simulink model "gm_sampleModel2052_3_sub"  (R2023a)
settings: Solver=VariableStepAuto  StartTime=0.0  StopTime=10.0  RelTol=1e-3
libraries: simulink x5, hdlsllib x1
settings Model: Creator=user1  LastModifiedBy=user1
settings OptimizationCC: BlockReduction=off  ConditionallyExecuteInputs=off
settings DebuggingCC: InheritedTsInSrcMsg=none

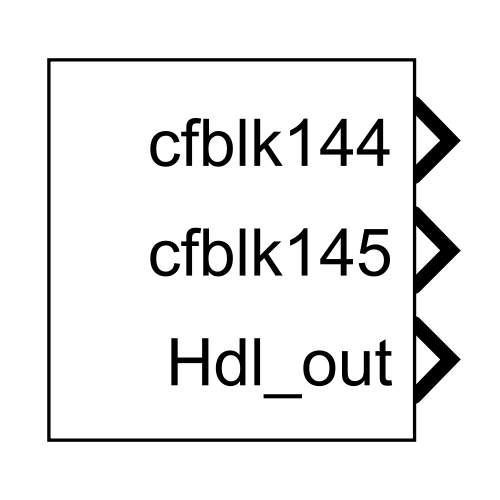
[thumbnail: Simulink's stored preview of the top-level diagram]
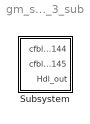
== system gm_sampleModel2052_3_sub ==
  Subsystem : Subsystem

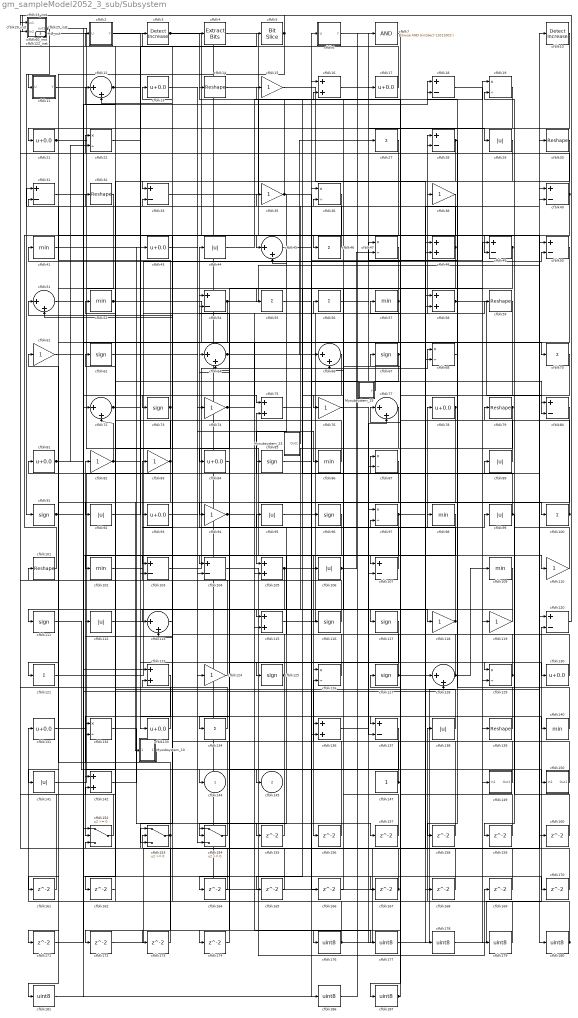
== system gm_sampleModel2052_3_sub/Subsystem ==
  Mysubsystem_10 : Subsystem
  Mysubsystem_15 : Subsystem
  Mysubsystem_23 : Subsystem
  cfblk10 : simulink/Logic and Bit Operations/Detect Increase  vinit=0.0  OutDataTypeStr=uint8
      settings: LibrarySourceBlock=|
      | hdlsllib/Logic and Bit
      | Operations/Detect
      | Increase
  cfblk{27,46,55..56,70,100,121,134} (8 alike) : Sum  Inputs=+  OutDataTypeStr=uint8
  cfblk{14,30,32,59,79,101,139} (7 alike) : Reshape
  cfblk{41,52,57,86,98,102,109,140} (8 alike) : MinMax  OutDataTypeStr=uint8
  cfblk{18,28,31,33,40,49..50,54,80,103..104,107,120,137} (14 alike) : Sum  Inputs=+-  OutDataTypeStr=uint8
  cfblk{16,48,58,75,105,115,123,136,142} (9 alike) : Sum  OutDataTypeStr=uint8
  cfblk{29,44,89,92,95,99,106,112,138,141} (10 alike) : Abs  OutDataTypeStr=uint8  SaturateOnIntegerOverflow=off
  cfblk108_inst : Subsystem
  cfblk11 : Subsystem  mask(Detect Fall Nonpositive){vinit=double(0), InputProcessing=Elements as channels (sample based), OutDataTypeStr=uint8}
      mask prompts: vinit "Simulink:masks:InitialCondition_MP"; InputProcessing "Simulink:masks:InputProcessing_MP"; OutDataTypeStr "Simulink:masks:OutputDataType_MP"
      mask help: Simulink:masks:DetectFallNonpositive_MD
      mask init:
      | InputProcessing = 'Elements as channels (sample based)';
      | OutDataTypeStr = 'uint8';
      | vinit = double(0);
      mask TypeOptions InputProcessing: Simulink:masks:ColumnsAsChannelsFrameBased | Simulink:masks:ElementsAsChannelsSampleBased
      mask TypeOptions OutDataTypeStr: Simulink:masks:uint8 | Simulink:masks:boolean
      mask Display: fprintf('U <= 0\n&  NOT\nU/z <= 0')
  cfblk{15,35,38,61,74,76,82..83,94,110,118..119,124} (13 alike) : Gain  OutDataTypeStr=uint8
  cfblk{62,67,73,85,91,96,111,116..117,125,127} (11 alike) : Signum
  cfblk{12,45,51,64,66,72,77,113,128} (9 alike) : Sum  Inputs=|++  OutDataTypeStr=uint8
  cfblk122_inst : Subsystem
  cfblk{19,22,36,47,68,87,97,126,129,132} (10 alike) : Product  Inputs=*/  OutDataTypeStr=uint8  RndMeth=Zero  SaturateOnIntegerOverflow=on
  cfblk{13,17,21,43,78,81,84,93,130..131,133} (11 alike) : Bias  Bias=0.0  SaturateOnIntegerOverflow=off
  cfblk147 : Constant  OutDataTypeStr=uint8  SampleTime=-1
  cfblk149 : Subsystem
  cfblk150 : Subsystem
  cfblk152 : Switch  OutDataTypeStr=uint8  SaturateOnIntegerOverflow=off  InputSameDT=off
  cfblk153 : Switch  OutDataTypeStr=uint8  SaturateOnIntegerOverflow=off  InputSameDT=off
  cfblk154 : Switch  OutDataTypeStr=uint8  SaturateOnIntegerOverflow=off  InputSameDT=off
  cfblk{155..162,164..174} (19 alike) : Delay  SampleTime=1
  cfblk{176..181,186..187} (8 alike) : DataTypeConversion  OutDataTypeStr=uint8  SaturateOnIntegerOverflow=off  RndMeth=Floor
  cfblk2 : Subsystem  mask(Detect Fall Nonpositive){vinit=double(0), InputProcessing=Elements as channels (sample based), OutDataTypeStr=uint8}
      mask prompts: vinit "Simulink:masks:InitialCondition_MP"; InputProcessing "Simulink:masks:InputProcessing_MP"; OutDataTypeStr "Simulink:masks:OutputDataType_MP"
      mask help: Simulink:masks:DetectFallNonpositive_MD
      mask init:
      | InputProcessing = 'Elements as channels (sample based)';
      | OutDataTypeStr = 'uint8';
      | vinit = double(0);
      mask TypeOptions InputProcessing: Simulink:masks:ColumnsAsChannelsFrameBased | Simulink:masks:ElementsAsChannelsSampleBased
      mask TypeOptions OutDataTypeStr: Simulink:masks:uint8 | Simulink:masks:boolean
      mask Display: fprintf('U <= 0\n&  NOT\nU/z <= 0')
  cfblk20_inst : Subsystem
  cfblk23_inst : Subsystem
  cfblk25_inst : Subsystem
  cfblk3 : simulink/Logic and Bit Operations/Detect Increase  vinit=0.0  OutDataTypeStr=uint8
      settings: LibrarySourceBlock=|
      | hdlsllib/Logic and Bit
      | Operations/Detect
      | Increase
  cfblk4 : simulink/Logic and Bit Operations/Extract Bits  bitsToExtract=Upper half  numBits=8  bitIdxRange=[0 7]  outScalingMode=Preserve fixed-point scaling
      settings: LibrarySourceBlock=|
      | hdlsllib/Logic and Bit
      | Operations/Extract Bits
  cfblk5 : hdlsllib/Logic and Bit Operations/Bit Slice  lidx=7  ridx=0
  cfblk6 : Subsystem  mask(Detect Rise Nonnegative){vinit=double(0), InputProcessing=Elements as channels (sample based), OutDataTypeStr=uint8}
      mask prompts: vinit "Simulink:masks:InitialCondition_MP"; InputProcessing "Simulink:masks:InputProcessing_MP"; OutDataTypeStr "Simulink:masks:OutputDataType_MP"
      mask help: Simulink:masks:DetectRiseNonnegative_MD
      mask init:
      | InputProcessing = 'Elements as channels (sample based)';
      | OutDataTypeStr = 'uint8';
      | vinit = double(0);
      mask TypeOptions InputProcessing: Simulink:masks:ColumnsAsChannelsFrameBased | Simulink:masks:ElementsAsChannelsSampleBased
      mask TypeOptions OutDataTypeStr: Simulink:masks:uint8 | Simulink:masks:boolean
      mask Display: fprintf('U >= 0\n&  NOT\nU/z >= 0')
  cfblk60_inst : Subsystem
  cfblk7 : simulink/Logic and Bit Operations/Bitwise Operator  logicop=AND  UseBitMask=on  BitMask=bin2dec('11011001')  BitMaskRealWorld=Stored Integer
      settings: LibrarySourceBlock=|
      | hdlsllib/Logic and Bit
      | Operations/Bitwise
      | Operator
  cfblk144 : Outport  OutDataTypeStr=uint8  SampleTime=1  VectorParamsAs1DForOutWhenUnconnected=off
  cfblk145 : Outport  Port=2  OutDataTypeStr=uint8  SampleTime=1  VectorParamsAs1DForOutWhenUnconnected=off
  Hdl_out : Outport  Port=3  OutDataTypeStr=uint8  SampleTime=1
  wires:
  Mysubsystem_10/1(Out1) -> cfblk82/1
  Mysubsystem_15/1(y) -> cfblk36/2
  Mysubsystem_23/1(Out1) -> cfblk33/2
  cfblk10/1 -> cfblk176/1
  cfblk100/1 -> cfblk79/1, cfblk41/1, cfblk57/1
  cfblk101/1 -> cfblk45/1
  cfblk102/1 -> cfblk50/2
  cfblk103/1 -> cfblk68/1
  cfblk104/1 -> cfblk169/1
  cfblk105/1 -> cfblk99/1, cfblk115/1
  cfblk106/1 -> cfblk17/1, cfblk47/2
  cfblk107/1 -> cfblk64/2
  cfblk108_inst/1(out1) -> cfblk105/1
  cfblk109/1 -> cfblk155/1
  cfblk11/1(Y) -> cfblk100/1
  cfblk110/1 -> cfblk89/1
  cfblk111/1 -> cfblk144/1
  cfblk112/1 -> cfblk56/1
  cfblk113/1 -> cfblk13/1
  cfblk115/1 -> cfblk28/1
  cfblk116/1 -> cfblk83/1
  cfblk117/1 -> cfblk164/1
  cfblk118/1 -> cfblk78/1, cfblk44/1
  cfblk119/1 -> cfblk117/1
  cfblk12/1 -> cfblk137/1, cfblk104/1
  cfblk120/1 -> cfblk122_inst/2(in2)
  cfblk121/1 -> cfblk98/1
  cfblk122_inst/1(out1) -> cfblk154/3, cfblk156/1
  cfblk123/1 -> cfblk152/2
  cfblk124/1 -> cfblk108_inst/2(in2)
  cfblk125/1 -> cfblk154/2, cfblk101/1
  cfblk126/1 -> cfblk51/1
  cfblk127/1 -> cfblk58/1, cfblk54/1
  cfblk128/1 -> cfblk77/1, cfblk109/1
  cfblk129/1 -> cfblk12/2, cfblk108_inst/1(in1)
  cfblk13/1 -> cfblk124/1
  cfblk130/1 -> cfblk95/1
  cfblk131/1 -> cfblk30/1
  cfblk132/1 -> cfblk157/1
  cfblk133/1 -> cfblk52/1
  cfblk134/1 -> cfblk20_inst/1(in1)
  cfblk136/1 -> cfblk97/1
  cfblk137/1 -> cfblk174/1
  cfblk138/1 -> cfblk62/1
  cfblk139/1 -> cfblk18/1
  cfblk14/1 -> cfblk166/1
  cfblk140/1 -> cfblk47/1
  cfblk141/1 -> cfblk75/2
  cfblk142/1 -> cfblk43/1
  cfblk147/1 -> cfblk66/2, cfblk20_inst/2(in2), cfblk87/1
  cfblk149/1(Out1) -> cfblk81/1
  cfblk15/1 -> cfblk128/1
  cfblk150/1(Out1) -> cfblk112/1
  cfblk152/1 -> cfblk25_inst/1(in1)
  cfblk153/1 -> cfblk61/1, cfblk172/1
  cfblk154/1 -> cfblk23_inst/2(in2)
  cfblk155/1 -> cfblk154/1
  cfblk156/1 -> cfblk126/2
  cfblk157/1 -> cfblk16/2
  cfblk158/1 -> cfblk51/2
  cfblk159/1 -> cfblk97/2
  cfblk16/1 -> cfblk29/1
  cfblk160/1 -> cfblk19/2
  cfblk161/1 -> cfblk60_inst/1(in1)
  cfblk162/1 -> cfblk142/2
  cfblk164/1 -> cfblk25_inst/2(in2)
  cfblk165/1 -> cfblk153/2
  cfblk166/1 -> cfblk136/1
  cfblk167/1 -> cfblk153/1, Hdl_out/1
  cfblk168/1 -> cfblk22/1
  cfblk169/1 -> cfblk152/1
  cfblk17/1 -> cfblk3/1
  cfblk170/1 -> cfblk123/2
  cfblk171/1 -> cfblk72/1
  cfblk172/1 -> cfblk40/2
  cfblk173/1 -> cfblk152/3
  cfblk174/1 -> cfblk64/1
  cfblk176/1 -> cfblk77/2, cfblk48/2, cfblk131/1, cfblk173/1
  cfblk177/1 -> cfblk10/1
  cfblk178/1 -> cfblk120/2
  cfblk179/1 -> cfblk2/1(U)
  cfblk18/1 -> cfblk149/1(In1)
  cfblk180/1 -> cfblk93/1, cfblk138/1, cfblk12/1
  cfblk181/1 -> cfblk6/1(U)
  cfblk186/1 -> cfblk7/1
  cfblk187/1 -> cfblk67/1, cfblk127/1
  cfblk19/1 -> cfblk21/1
  cfblk2/1(Y) -> cfblk178/1
  cfblk20_inst/1(out1) -> cfblk91/1, cfblk75/1
  cfblk21/1 -> cfblk129/2, cfblk46/1
  cfblk22/1 -> cfblk133/1
  cfblk23_inst/1(out1) -> cfblk128/2
  cfblk25_inst/1(out1) -> cfblk11/1(U), cfblk70/1
  cfblk27/1 -> cfblk85/1
  cfblk28/1 -> cfblk158/1, cfblk132/2
  cfblk29/1 -> cfblk33/1
  cfblk3/1 -> cfblk120/1, cfblk68/2
  cfblk30/1 -> cfblk58/2
  cfblk31/1 -> cfblk119/1
  cfblk32/1 -> cfblk171/1
  cfblk33/1 -> cfblk19/1
  cfblk35/1 -> cfblk45/2, cfblk4/1, cfblk110/1
  cfblk36/1 -> cfblk181/1
  cfblk38/1 -> cfblk162/1
  cfblk4/1 -> cfblk49/2
  cfblk40/1 -> cfblk23_inst/1(in1), cfblk153/3
  cfblk41/1 -> cfblk179/1
  cfblk43/1 -> cfblk74/1
  cfblk44/1 -> cfblk16/1
  cfblk45/1 -> cfblk66/1
  cfblk46/1 -> cfblk36/1
  cfblk47/1 -> cfblk116/1
  cfblk48/1 -> cfblk84/1, cfblk32/1, cfblk35/1
  cfblk49/1 -> cfblk76/1, cfblk165/1
  cfblk5/1 -> cfblk141/1, cfblk122_inst/1(in1)
  cfblk50/1 -> cfblk161/1
  cfblk51/1 -> cfblk123/1
  cfblk52/1 -> cfblk115/2, cfblk168/1
  cfblk54/1 -> cfblk50/1, cfblk48/1, cfblk103/1
  cfblk55/1 -> cfblk96/1
  cfblk56/1 -> cfblk139/1
  cfblk57/1 -> cfblk136/2, cfblk55/1
  cfblk58/1 -> cfblk80/2, cfblk28/2, cfblk160/1
  cfblk59/1 -> cfblk107/1
  cfblk6/1(Y) -> cfblk180/1
  cfblk60_inst/1(out1) -> cfblk73/1
  cfblk61/1 -> cfblk186/1
  cfblk62/1 -> cfblk86/1
  cfblk64/1 -> cfblk80/1, cfblk27/1
  cfblk66/1 -> cfblk145/1
  cfblk67/1 -> cfblk92/1, cfblk87/2
  cfblk68/1 -> cfblk38/1
  cfblk7/1 -> cfblk187/1
  cfblk70/1 -> cfblk106/1
  cfblk72/1 -> cfblk129/1, cfblk118/1
  cfblk73/1 -> cfblk31/2, cfblk142/1
  cfblk74/1 -> cfblk59/1, cfblk126/1
  cfblk75/1 -> cfblk167/1
  cfblk76/1 -> cfblk140/1
  cfblk77/1 -> cfblk111/1
  cfblk78/1 -> cfblk113/1, cfblk103/2
  cfblk79/1 -> cfblk105/2, cfblk94/1
  cfblk80/1 -> cfblk113/2
  cfblk81/1 -> cfblk104/2, cfblk22/2
  cfblk82/1 -> cfblk72/2, cfblk107/2
  cfblk83/1 -> cfblk31/1, Mysubsystem_10/1(In1)
  cfblk84/1 -> cfblk134/1
  cfblk85/1 -> cfblk137/2
  cfblk86/1 -> cfblk60_inst/2(in2)
  cfblk87/1 -> cfblk121/1
  cfblk89/1 -> cfblk14/1
  cfblk91/1 -> cfblk18/2, cfblk170/1, cfblk150/1(In1)
  cfblk92/1 -> cfblk5/1
  cfblk93/1 -> cfblk130/1
  cfblk94/1 -> cfblk54/2, cfblk177/1
  cfblk95/1 -> cfblk49/1
  cfblk96/1 -> cfblk132/1
  cfblk97/1 -> cfblk40/1, cfblk125/1
  cfblk98/1 -> cfblk102/1
  cfblk99/1 -> cfblk159/1, cfblk15/1

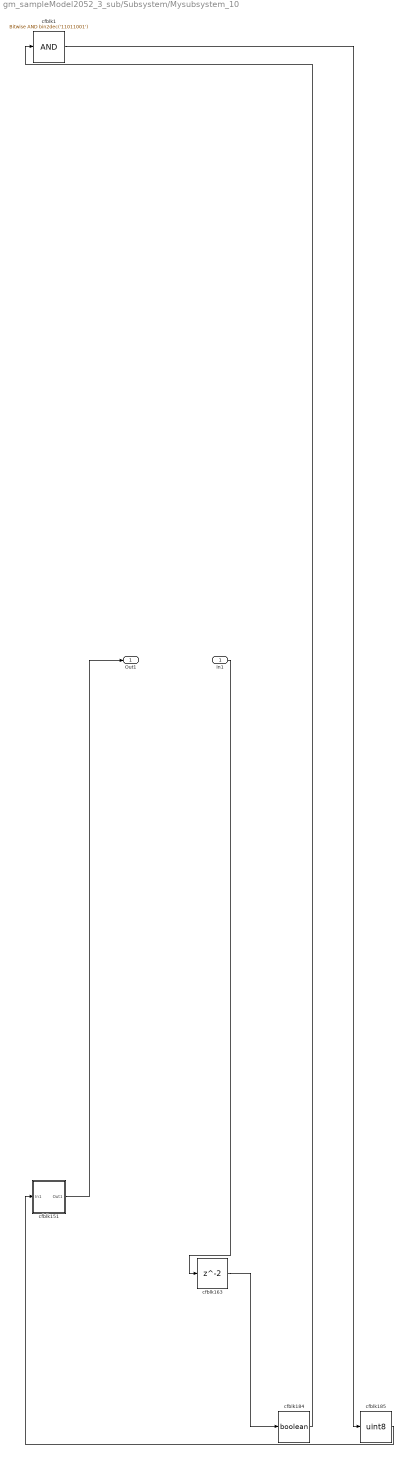
== system gm_sampleModel2052_3_sub/Subsystem/Mysubsystem_10 ==
  In1 : Inport  OutDataTypeStr=uint8  PortDimensions=1  SampleTime=1
  cfblk1 : simulink/Logic and Bit Operations/Bitwise Operator  logicop=AND  UseBitMask=on  BitMask=bin2dec('11011001')  BitMaskRealWorld=Stored Integer
      settings: LibrarySourceBlock=|
      | hdlsllib/Logic and Bit
      | Operations/Bitwise
      | Operator
  cfblk151 : Subsystem
  cfblk163 : Delay  SampleTime=1
  cfblk184 : DataTypeConversion  OutDataTypeStr=boolean  SaturateOnIntegerOverflow=off  RndMeth=Floor
  cfblk185 : DataTypeConversion  OutDataTypeStr=uint8  SaturateOnIntegerOverflow=off  RndMeth=Floor
  Out1 : Outport  SampleTime=1
  wires:
  In1/1 -> cfblk163/1
  cfblk1/1 -> cfblk185/1
  cfblk151/1(Out1) -> Out1/1
  cfblk163/1 -> cfblk184/1
  cfblk184/1 -> cfblk1/1
  cfblk185/1 -> cfblk151/1(In1)

== system gm_sampleModel2052_3_sub/Subsystem/Mysubsystem_15 ==
  cfblk148 : Subsystem  mask(Counter Free-Running){NumBits=double(16), tsamp=double(-1)}
      mask prompts: NumBits "Simulink:masks:NumberOfBits_MP"; tsamp "Simulink:masks:SampleTime_MP"
      mask help: Simulink:masks:CounterFreeRunning_MD
  y : Outport  SampleTime=1
  wires:
  cfblk148/1(y) -> y/1

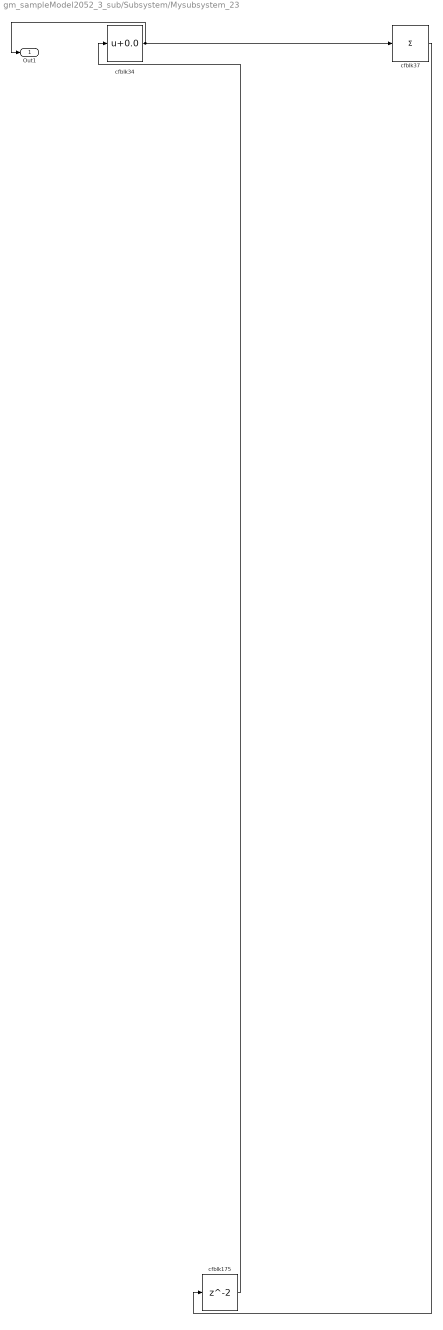
== system gm_sampleModel2052_3_sub/Subsystem/Mysubsystem_23 ==
  cfblk175 : Delay  SampleTime=1
  cfblk34 : Bias  Bias=0.0  SaturateOnIntegerOverflow=off
  cfblk37 : Sum  Inputs=+
  Out1 : Outport  SampleTime=1
  wires:
  cfblk175/1 -> cfblk34/1
  cfblk34/1 -> Out1/1, cfblk37/1
  cfblk37/1 -> cfblk175/1

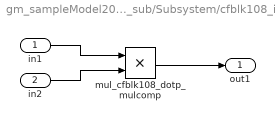
== system gm_sampleModel2052_3_sub/Subsystem/cfblk108_inst ==
  in1 : Inport  OutDataTypeStr=uint8  SampleTime=1
  in2 : Inport  Port=2  OutDataTypeStr=uint8  SampleTime=1
  mul_cfblk108_dotp_mulcomp : Product  Inputs=**  OutDataTypeStr=uint8  SampleTime=1
  out1 : Outport  OutDataTypeStr=uint8  SampleTime=1
  wires:
  in1/1 -> mul_cfblk108_dotp_mulcomp/1
  in2/1 -> mul_cfblk108_dotp_mulcomp/2
  mul_cfblk108_dotp_mulcomp/1 -> out1/1

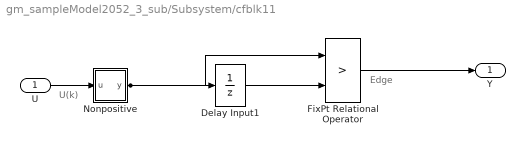
== system gm_sampleModel2052_3_sub/Subsystem/cfblk11 ==
  note: U(k)
  note: Edge
  U : Inport  OutDataTypeStr=uint8  SampleTime=1
  Delay Input1 : UnitDelay  Description=Store in Global RAM  DisableCoverage=on  InitialCondition=vinit  SampleTime=-1  HasFrameUpgradeWarning=on
  FixPt Relational Operator : RelationalOperator  Operator=>  OutDataTypeStr=fixdt(0, 8)  ZeroCross=off  InputSameDT=off
  Nonpositive : Subsystem  mask(Compare To Zero){relop=<=, OutDataTypeStr=boolean, ZeroCross=off}
      mask prompts: relop "Simulink:masks:Operator_MP"; OutDataTypeStr "Simulink:masks:OutputDataType_MP"; ZeroCross "Simulink:masks:EnableZerocrossingDetection_MP"
      mask help: Simulink:masks:CompareToZero_MD
      mask init:
      | OutDataTypeStr = 'boolean';
      | ZeroCross = 'off';
      | blkName = 'sampleModel2052_3_sub/Subsystem/cfblk11/Nonpositive';
      | relop = '<=';
      | setValue = 'boolean';
      mask TypeOptions relop: == | ~= | < | <= | >= | >
      mask TypeOptions OutDataTypeStr: Simulink:masks:uint8 | Simulink:masks:boolean
      mask Callback ZeroCross: sl('zeroCrossEnable', gcbh);
      mask Display: disp([relop,' 0'])
  Y : Outport  SampleTime=1
  wires:
  U/1 -> Nonpositive/1(u)
  Delay Input1/1 -> FixPt Relational Operator/2
  FixPt Relational Operator/1 -> Y/1
  Nonpositive/1(y) -> FixPt Relational Operator/1, Delay Input1/1

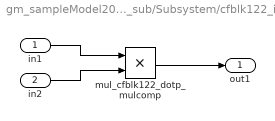
== system gm_sampleModel2052_3_sub/Subsystem/cfblk122_inst ==
  in1 : Inport  OutDataTypeStr=uint8  SampleTime=1
  in2 : Inport  Port=2  OutDataTypeStr=uint8  SampleTime=1
  mul_cfblk122_dotp_mulcomp : Product  Inputs=**  OutDataTypeStr=uint8  SampleTime=1
  out1 : Outport  OutDataTypeStr=uint8  SampleTime=1
  wires:
  in1/1 -> mul_cfblk122_dotp_mulcomp/1
  in2/1 -> mul_cfblk122_dotp_mulcomp/2
  mul_cfblk122_dotp_mulcomp/1 -> out1/1

== system gm_sampleModel2052_3_sub/Subsystem/cfblk149 ==
  In1 : Inport  OutDataTypeStr=uint8  PortDimensions=1  SampleTime=1
  Out1 : Outport  SampleTime=1
  wires:
  In1/1 -> Out1/1

== system gm_sampleModel2052_3_sub/Subsystem/cfblk150 ==
  In1 : Inport  OutDataTypeStr=uint8  PortDimensions=1  SampleTime=1
  Out1 : Outport  SampleTime=1
  wires:
  In1/1 -> Out1/1

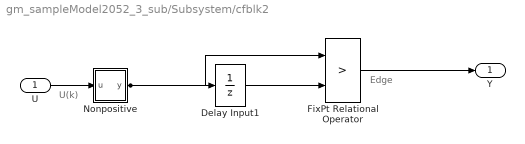
== system gm_sampleModel2052_3_sub/Subsystem/cfblk2 ==
  note: U(k)
  note: Edge
  U : Inport  OutDataTypeStr=uint8  SampleTime=1
  Delay Input1 : UnitDelay  Description=Store in Global RAM  DisableCoverage=on  InitialCondition=vinit  SampleTime=-1  HasFrameUpgradeWarning=on
  FixPt Relational Operator : RelationalOperator  Operator=>  OutDataTypeStr=fixdt(0, 8)  ZeroCross=off  InputSameDT=off
  Nonpositive : Subsystem  mask(Compare To Zero){relop=<=, OutDataTypeStr=boolean, ZeroCross=off}
      mask prompts: relop "Simulink:masks:Operator_MP"; OutDataTypeStr "Simulink:masks:OutputDataType_MP"; ZeroCross "Simulink:masks:EnableZerocrossingDetection_MP"
      mask help: Simulink:masks:CompareToZero_MD
      mask init:
      | OutDataTypeStr = 'boolean';
      | ZeroCross = 'off';
      | blkName = 'sampleModel2052_3_sub/Subsystem/cfblk2/Nonpositive';
      | relop = '<=';
      | setValue = 'boolean';
      mask TypeOptions relop: == | ~= | < | <= | >= | >
      mask TypeOptions OutDataTypeStr: Simulink:masks:uint8 | Simulink:masks:boolean
      mask Callback ZeroCross: sl('zeroCrossEnable', gcbh);
      mask Display: disp([relop,' 0'])
  Y : Outport  SampleTime=1
  wires:
  U/1 -> Nonpositive/1(u)
  Delay Input1/1 -> FixPt Relational Operator/2
  FixPt Relational Operator/1 -> Y/1
  Nonpositive/1(y) -> FixPt Relational Operator/1, Delay Input1/1

== system gm_sampleModel2052_3_sub/Subsystem/cfblk20_inst ==
  in1 : Inport  OutDataTypeStr=uint8  SampleTime=1
  in2 : Inport  Port=2  OutDataTypeStr=uint8  SampleTime=1
  mul_cfblk20_dotp_mulcomp : Product  Inputs=**  OutDataTypeStr=uint8  SampleTime=1
  out1 : Outport  OutDataTypeStr=uint8  SampleTime=1
  wires:
  in1/1 -> mul_cfblk20_dotp_mulcomp/1
  in2/1 -> mul_cfblk20_dotp_mulcomp/2
  mul_cfblk20_dotp_mulcomp/1 -> out1/1

== system gm_sampleModel2052_3_sub/Subsystem/cfblk23_inst ==
  in1 : Inport  OutDataTypeStr=uint8  SampleTime=1
  in2 : Inport  Port=2  OutDataTypeStr=uint8  SampleTime=1
  mul_cfblk23_dotp_mulcomp : Product  Inputs=**  OutDataTypeStr=uint8  SampleTime=1
  out1 : Outport  OutDataTypeStr=uint8  SampleTime=1
  wires:
  in1/1 -> mul_cfblk23_dotp_mulcomp/1
  in2/1 -> mul_cfblk23_dotp_mulcomp/2
  mul_cfblk23_dotp_mulcomp/1 -> out1/1

== system gm_sampleModel2052_3_sub/Subsystem/cfblk25_inst ==
  in1 : Inport  OutDataTypeStr=uint8  SampleTime=1
  in2 : Inport  Port=2  OutDataTypeStr=uint8  SampleTime=1
  mul_cfblk25_dotp_mulcomp : Product  Inputs=**  OutDataTypeStr=uint8  SampleTime=1
  out1 : Outport  OutDataTypeStr=uint8  SampleTime=1
  wires:
  in1/1 -> mul_cfblk25_dotp_mulcomp/1
  in2/1 -> mul_cfblk25_dotp_mulcomp/2
  mul_cfblk25_dotp_mulcomp/1 -> out1/1

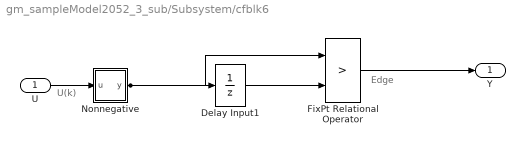
== system gm_sampleModel2052_3_sub/Subsystem/cfblk6 ==
  note: U(k)
  note: Edge
  U : Inport  OutDataTypeStr=uint8  SampleTime=1
  Delay Input1 : UnitDelay  Description=Store in Global RAM  DisableCoverage=on  InitialCondition=vinit  SampleTime=-1  HasFrameUpgradeWarning=on
  FixPt Relational Operator : RelationalOperator  Operator=>  OutDataTypeStr=fixdt(0, 8)  ZeroCross=off  InputSameDT=off
  Nonnegative : Subsystem  mask(Compare To Zero){relop=>=, OutDataTypeStr=boolean, ZeroCross=off}
      mask prompts: relop "Simulink:masks:Operator_MP"; OutDataTypeStr "Simulink:masks:OutputDataType_MP"; ZeroCross "Simulink:masks:EnableZerocrossingDetection_MP"
      mask help: Simulink:masks:CompareToZero_MD
      mask init:
      | OutDataTypeStr = 'boolean';
      | ZeroCross = 'off';
      | blkName = 'sampleModel2052_3_sub/Subsystem/cfblk6/Nonnegative';
      | relop = '>=';
      | setValue = 'boolean';
      mask TypeOptions relop: == | ~= | < | <= | >= | >
      mask TypeOptions OutDataTypeStr: Simulink:masks:uint8 | Simulink:masks:boolean
      mask Callback ZeroCross: sl('zeroCrossEnable', gcbh);
      mask Display: disp([relop,' 0'])
  Y : Outport  SampleTime=1
  wires:
  U/1 -> Nonnegative/1(u)
  Delay Input1/1 -> FixPt Relational Operator/2
  FixPt Relational Operator/1 -> Y/1
  Nonnegative/1(y) -> FixPt Relational Operator/1, Delay Input1/1

== system gm_sampleModel2052_3_sub/Subsystem/cfblk60_inst ==
  in1 : Inport  OutDataTypeStr=uint8  SampleTime=1
  in2 : Inport  Port=2  OutDataTypeStr=uint8  SampleTime=1
  mul_cfblk60_dotp_mulcomp : Product  Inputs=**  OutDataTypeStr=uint8  SampleTime=1
  out1 : Outport  OutDataTypeStr=uint8  SampleTime=1
  wires:
  in1/1 -> mul_cfblk60_dotp_mulcomp/1
  in2/1 -> mul_cfblk60_dotp_mulcomp/2
  mul_cfblk60_dotp_mulcomp/1 -> out1/1

== system gm_sampleModel2052_3_sub/Subsystem/Mysubsystem_10/cfblk151 ==
  In1 : Inport  OutDataTypeStr=uint8  PortDimensions=1  SampleTime=1
  Out1 : Outport  SampleTime=1
  wires:
  In1/1 -> Out1/1

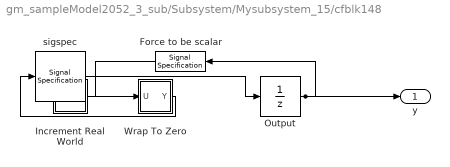
== system gm_sampleModel2052_3_sub/Subsystem/Mysubsystem_15/cfblk148 ==
  Force to be scalar : SignalSpecification  DisableCoverage=on  Dimensions=1
  Increment Real World : Subsystem  mask(Real World Value Increment){}
      mask help: Simulink:masks:RealWorldValueIncrement_MD
      mask Display: disp('V++')
  Output : UnitDelay  InitialCondition=0.0  SampleTime=tsamp  HasFrameUpgradeWarning=on
  Wrap To Zero : Subsystem  mask(Wrap To Zero){Threshold=double(65535)}
      mask prompts: Threshold "Simulink:masks:Threshold_MP"
      mask help: Simulink:masks:WrapToZero_MD
  sigspec : SignalSpecification  OutDataTypeStr=uint16  Dimensions=1
  y : Outport  SampleTime=1
  wires:
  Force to be scalar/1 -> Increment Real World/1(u)
  Increment Real World/1(y) -> Wrap To Zero/1(U)
  Output/1 -> Force to be scalar/1, y/1
  Wrap To Zero/1(Y) -> sigspec/1
  sigspec/1 -> Output/1

== system gm_sampleModel2052_3_sub/Subsystem/cfblk11/Nonpositive ==
  u : Inport  OutDataTypeStr=uint8  SampleTime=1
  Compare : RelationalOperator  Operator=<=  OutDataTypeStr=boolean  ZeroCross=off
  Constant : Constant  DisableCoverage=on  Value=0  OutDataTypeStr=Inherit: Inherit via back propagation  SampleTime=-1  PreserveConstantTs=on
  y : Outport  SampleTime=1
  wires:
  u/1 -> Compare/1
  Compare/1 -> y/1
  Constant/1 -> Compare/2

== system gm_sampleModel2052_3_sub/Subsystem/cfblk2/Nonpositive ==
  u : Inport  OutDataTypeStr=uint8  SampleTime=1
  Compare : RelationalOperator  Operator=<=  OutDataTypeStr=boolean  ZeroCross=off
  Constant : Constant  DisableCoverage=on  Value=0  OutDataTypeStr=Inherit: Inherit via back propagation  SampleTime=-1  PreserveConstantTs=on
  y : Outport  SampleTime=1
  wires:
  u/1 -> Compare/1
  Compare/1 -> y/1
  Constant/1 -> Compare/2

== system gm_sampleModel2052_3_sub/Subsystem/cfblk6/Nonnegative ==
  u : Inport  OutDataTypeStr=uint8  SampleTime=1
  Compare : RelationalOperator  OutDataTypeStr=boolean  ZeroCross=off
  Constant : Constant  DisableCoverage=on  Value=0  OutDataTypeStr=Inherit: Inherit via back propagation  SampleTime=-1  PreserveConstantTs=on
  y : Outport  SampleTime=1
  wires:
  u/1 -> Compare/1
  Compare/1 -> y/1
  Constant/1 -> Compare/2

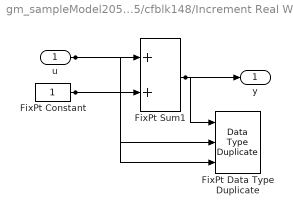
== system gm_sampleModel2052_3_sub/Subsystem/Mysubsystem_15/cfblk148/Increment Real World ==
  u : Inport  OutDataTypeStr=uint16  SampleTime=1
  FixPt Constant : Constant  DisableCoverage=on  OutDataTypeStr=Inherit: Inherit via back propagation  SampleTime=-1
  FixPt Data Type Duplicate : DataTypeDuplicate  DisableCoverage=on  NumInputPorts=3
  FixPt Sum1 : Sum  InputSameDT=on  OutDataTypeStr=Inherit: Inherit via back propagation  LockScale=on
  y : Outport  SampleTime=1
  wires:
  u/1 -> FixPt Sum1/1, FixPt Data Type Duplicate/2
  FixPt Constant/1 -> FixPt Sum1/2, FixPt Data Type Duplicate/3
  FixPt Sum1/1 -> FixPt Data Type Duplicate/1, y/1

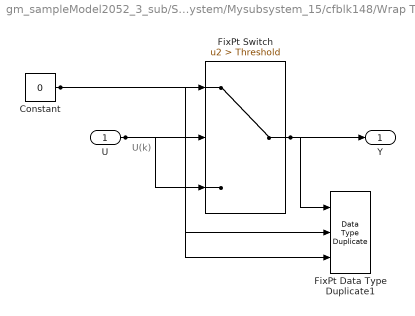
== system gm_sampleModel2052_3_sub/Subsystem/Mysubsystem_15/cfblk148/Wrap To Zero ==
  note: U(k)
  U : Inport  OutDataTypeStr=uint16  SampleTime=1
  Constant : Constant  DisableCoverage=on  Value=0  OutDataTypeStr=Inherit: Inherit via back propagation  SampleTime=-1
  FixPt Data Type Duplicate1 : DataTypeDuplicate  DisableCoverage=on  NumInputPorts=3
  FixPt Switch : Switch  Criteria=u2 > Threshold  Threshold=Threshold  OutDataTypeStr=Inherit: Inherit via back propagation  ZeroCross=off  SaturateOnIntegerOverflow=off  InputSameDT=off
  Y : Outport  SampleTime=1
  wires:
  U/1 -> FixPt Switch/3, FixPt Switch/2, FixPt Data Type Duplicate1/2
  Constant/1 -> FixPt Switch/1, FixPt Data Type Duplicate1/3
  FixPt Switch/1 -> FixPt Data Type Duplicate1/1, Y/1
